simulink model "trajectoryReplay"  (R2018b)
settings: configuration reference "Physics" (kept outside this file)
StartFcn:
  | dictObj = Simulink.data.dictionary.open('ScenarioDefinition.sldd');
  | secObj = getSection(dictObj, 'Design Data');
  | enObj = getEntry(secObj, 'Raceline_Op1');
  | temp = getValue(enObj);
  | set_param('trajectoryReplay/max_v_Op1','Value',num2str(max(temp.vx_mps)));
  | 
  | close(dictObj);
  | clear dictObj secObj enObj temp;
model workspace (MAT data in the model file):
  F_N_Op = Simulink.Parameter
  F_N_Op.Value = [1 2 3 4 5 6 7 8 9 10 11 12 ... (5000 elements, 5000x1)]
  F_N_Op.DataType = 'auto'
  F_N_Op.Dimensions = [5000 1]
  ValidPointCnt_Op = 4844
  ax_mps2_Op = Simulink.Parameter
  ax_mps2_Op.Value = [1 2 3 4 5 6 7 8 9 10 11 12 ... (5000 elements, 5000x1)]
  ax_mps2_Op.DataType = 'auto'
  ax_mps2_Op.Dimensions = [5000 1]
  dPsi_radps = Simulink.Parameter
  dPsi_radps.Value = 0
  dPsi_radps.DataType = 'auto'
  dPsi_radps.Dimensions = [1 1]
  delta_rad_Op = Simulink.Parameter
  delta_rad_Op.Value = [1 2 3 4 5 6 7 8 9 10 11 12 ... (5000 elements, 5000x1)]
  delta_rad_Op.DataType = 'auto'
  delta_rad_Op.Dimensions = [5000 1]
  kappa_radpm_Op = Simulink.Parameter
  kappa_radpm_Op.Value = [1 2 3 4 5 6 7 8 9 10 11 12 ... (5000 elements, 5000x1)]
  kappa_radpm_Op.DataType = 'auto'
  kappa_radpm_Op.Dimensions = [5000 1]
  psi0_rad = Simulink.Parameter
  psi0_rad.Value = 0
  psi0_rad.DataType = 'auto'
  psi0_rad.Dimensions = [1 1]
  psi_rad = Simulink.Parameter
  psi_rad.Value = 0
  psi_rad.DataType = 'auto'
  psi_rad.Dimensions = [1 1]
  psi_rad_Op = Simulink.Parameter
  psi_rad_Op.Value = [1 2 3 4 5 6 7 8 9 10 11 12 ... (5000 elements, 5000x1)]
  psi_rad_Op.DataType = 'auto'
  psi_rad_Op.Dimensions = [5000 1]
  s0_m = Simulink.Parameter
  s0_m.Value = 0
  s0_m.DataType = 'auto'
  s0_m.Dimensions = [1 1]
  s_m_Op = Simulink.Parameter
  s_m_Op.Value = [1 2 3 4 5 6 7 8 9 10 11 12 ... (5000 elements, 5000x1)]
  s_m_Op.DataType = 'auto'
  s_m_Op.Dimensions = [5000 1]
  s_m_end_Op = Simulink.Parameter
  s_m_end_Op.Value = 0
  s_m_end_Op.DataType = 'double'
  s_m_end_Op.Dimensions = [1 1]
  velGain_Op = Simulink.Parameter
  velGain_Op.Value = 0
  velGain_Op.DataType = 'auto'
  velGain_Op.Dimensions = [1 1]
  vx_mps = Simulink.Parameter
  vx_mps.Value = 0
  vx_mps.DataType = 'auto'
  vx_mps.Dimensions = [1 1]
  vx_mps_Op = Simulink.Parameter
  vx_mps_Op.Value = [1 2 3 4 5 6 7 8 9 10 11 12 ... (5000 elements, 5000x1)]
  vx_mps_Op.DataType = 'auto'
  vx_mps_Op.Dimensions = [5000 1]
  vy_mps = Simulink.Parameter
  vy_mps.Value = 0
  vy_mps.DataType = 'auto'
  vy_mps.Dimensions = [1 1]
  x0_m = Simulink.Parameter
  x0_m.Value = 0
  x0_m.DataType = 'auto'
  x0_m.Dimensions = [1 1]
  x0_vehiclepose_Op = Simulink.Parameter
  x0_vehiclepose_Op.Value = [0 0 0]
  x0_vehiclepose_Op.DataType = 'double'
  x0_vehiclepose_Op.Dimensions = [1 3]
  x_m = Simulink.Parameter
  x_m.Value = 0
  x_m.DataType = 'double'
  x_m.Dimensions = [1 1]
  x_m_Op = Simulink.Parameter
  x_m_Op.Value = [1 2 3 4 5 6 7 8 9 10 11 12 ... (5000 elements, 5000x1)]
  x_m_Op.DataType = 'auto'
  x_m_Op.Dimensions = [5000 1]
  y0_m = Simulink.Parameter
  y0_m.Value = 0
  y0_m.DataType = 'auto'
  y0_m.Dimensions = [1 1]
  y_m = Simulink.Parameter
  y_m.Value = 0
  y_m.DataType = 'double'
  y_m.Dimensions = [1 1]
  y_m_Op = Simulink.Parameter
  y_m_Op.Value = [1 2 3 4 5 6 7 8 9 10 11 12 ... (5000 elements, 5000x1)]
  y_m_Op.DataType = 'auto'
  y_m_Op.Dimensions = [5000 1]
undefined symbols (not defined in the file): tSSlow
libraries: simulink x1
settings Model: DataDictionary=trajectoryReplay.sldd  ParameterArgumentNames=F_N_Op,ValidPointCnt_Op,ax_mps2_Op,delta_rad_Op,kappa_radpm_Op,psi_rad_Op,s0_m,s_m_Op,s_m_end_Op,velGain_Op,vx_mps_Op,x0_vehiclepose_Op,x_m_Op,y_m_Op  OrderedModelArguments=off  Creator=wischnewski  LastModifiedBy=ge34qer

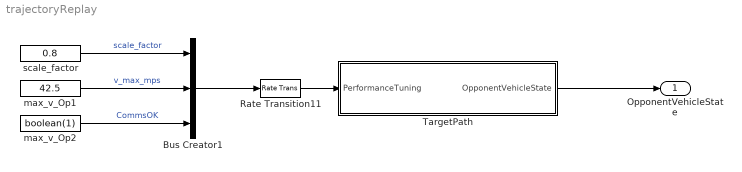
== system trajectoryReplay ==
  Bus Creator1 : BusCreator  Inputs=3  OutDataTypeStr=Bus: Planning_ControlPerformance_Feedback
  Rate Transition11 : RateTransition
  TargetPath : Subsystem  SystemSampleTime=tSSlow
  max_v_Op1 : Constant  Value=42.5
  max_v_Op2 : Constant  Value=boolean(1)
  scale_factor : Constant  Value=0.8
  OpponentVehicleState : Outport  OutDataTypeStr=Bus: V2X_Vehicle_Sim
  wires:
  Rate Transition11/1 -> TargetPath/1(PerformanceTuning)
  scale_factor/1 -> Bus Creator1/1  "scale_factor"
  max_v_Op1/1 -> Bus Creator1/2  "v_max_mps"
  Bus Creator1/1 -> Rate Transition11/1
  max_v_Op2/1 -> Bus Creator1/3  "CommsOK"
  TargetPath/1(OpponentVehicleState) -> OpponentVehicleState/1

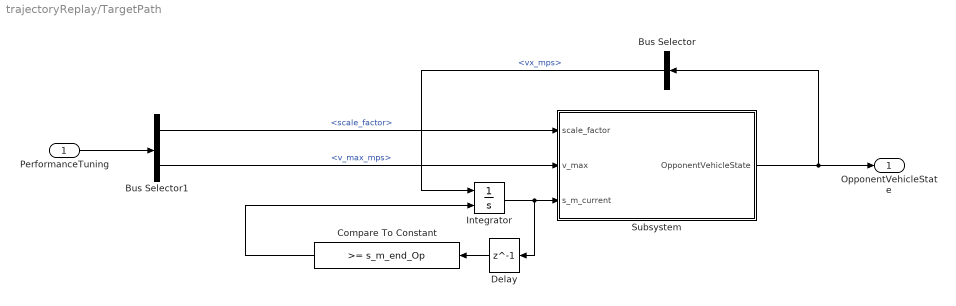
== system trajectoryReplay/TargetPath ==
  PerformanceTuning : Inport  OutDataTypeStr=Bus: Planning_ControlPerformance_Feedback
  Bus Selector : BusSelector  OutputSignals=vx_mps
  Bus Selector1 : BusSelector  OutputSignals=scale_factor,v_max_mps
  Compare To Constant : simulink/Logic and Bit Operations/Compare To Constant  relop=>=  const=s_m_end_Op  OutDataTypeStr=boolean
  Delay : Delay  DelayLength=1
  Integrator : Integrator  ExternalReset=rising  InitialCondition=s0_m
  Subsystem : Subsystem
  OpponentVehicleState : Outport
  wires:
  Integrator/1 -> Delay/1, Subsystem/3(s_m_current)
  Delay/1 -> Compare To Constant/1
  Subsystem/1(OpponentVehicleState) -> OpponentVehicleState/1, Bus Selector/1
  Compare To Constant/1 -> Integrator/2
  PerformanceTuning/1 -> Bus Selector1/1
  Bus Selector1/1 -> Subsystem/1(scale_factor)  "<scale_factor>"
  Bus Selector1/2 -> Subsystem/2(v_max)  "<v_max_mps>"
  Bus Selector/1 -> Integrator/1  "<vx_mps>"

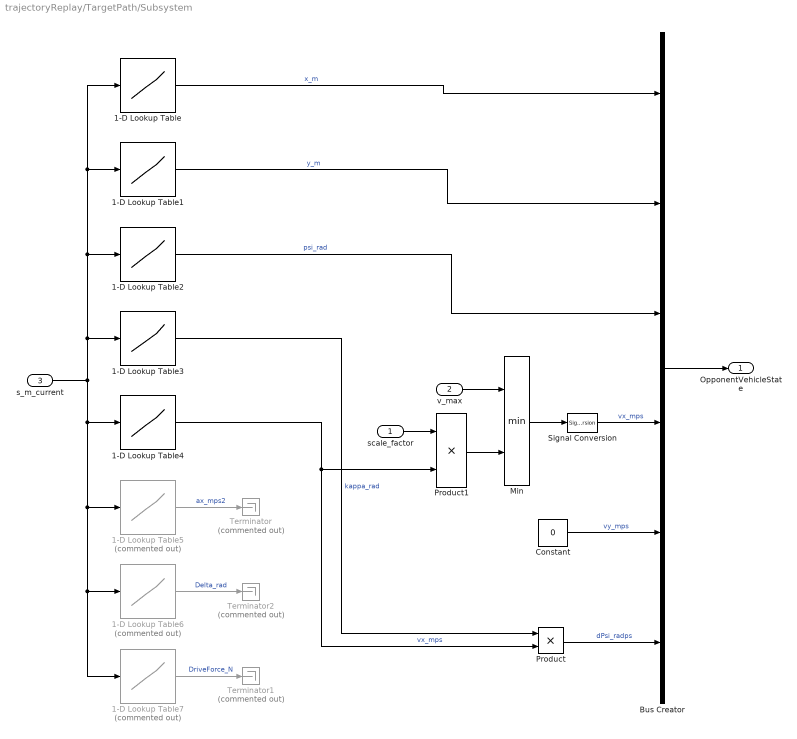
== system trajectoryReplay/TargetPath/Subsystem ==
  scale_factor : Inport
  v_max : Inport  Port=2
  s_m_current : Inport  Port=3
  1-D Lookup Table : Lookup_n-D  NumberOfTableDimensions=1  BreakpointsForDimension1=s_m_Op  Table=x_m_Op  InternalRulePriority=Speed  RndMeth=Simplest  InputSameDT=on
  1-D Lookup Table1 : Lookup_n-D  NumberOfTableDimensions=1  BreakpointsForDimension1=s_m_Op  Table=y_m_Op  InternalRulePriority=Speed  RndMeth=Simplest  InputSameDT=on
  1-D Lookup Table2 : Lookup_n-D  NumberOfTableDimensions=1  BreakpointsForDimension1=s_m_Op  Table=psi_rad_Op  InternalRulePriority=Speed  RndMeth=Simplest  InputSameDT=on
  1-D Lookup Table3 : Lookup_n-D  NumberOfTableDimensions=1  BreakpointsForDimension1=s_m_Op  Table=kappa_radpm_Op  InternalRulePriority=Speed  RndMeth=Simplest  InputSameDT=on
  1-D Lookup Table4 : Lookup_n-D  NumberOfTableDimensions=1  BreakpointsForDimension1=s_m_Op  Table=vx_mps_Op  InternalRulePriority=Speed  RndMeth=Simplest  InputSameDT=on
  1-D Lookup Table5 : Lookup_n-D  Commented=on  NumberOfTableDimensions=1  BreakpointsForDimension1=s_m_Op  Table=ax_mps2_Op  InternalRulePriority=Speed  RndMeth=Simplest  InputSameDT=on
  1-D Lookup Table6 : Lookup_n-D  Commented=on  NumberOfTableDimensions=1  BreakpointsForDimension1=s_m_Op  Table=delta_rad_Op  InternalRulePriority=Speed  RndMeth=Simplest  InputSameDT=on
  1-D Lookup Table7 : Lookup_n-D  Commented=on  NumberOfTableDimensions=1  BreakpointsForDimension1=s_m_Op  Table=F_N_Op  InternalRulePriority=Speed  RndMeth=Simplest  InputSameDT=on
  Bus Creator : BusCreator  Inputs=6  OutDataTypeStr=Bus: V2X_Vehicle_Sim
  Constant : Constant  Value=0
  Min : MinMax  Inputs=2
  Product : Product
  Product1 : Product
  Signal Conversion : SignalConversion  OverrideOpt=off
  Terminator : Terminator  Commented=on
  Terminator1 : Terminator  Commented=on
  Terminator2 : Terminator  Commented=on
  OpponentVehicleState : Outport
  wires:
  1-D Lookup Table6/1 -> Terminator2/1  "Delta_rad"
  1-D Lookup Table/1 -> Bus Creator/1  "x_m"
  s_m_current/1 -> 1-D Lookup Table/1, 1-D Lookup Table1/1, 1-D Lookup Table2/1, 1-D Lookup Table3/1, 1-D Lookup Table7/1, 1-D Lookup Table6/1, 1-D Lookup Table5/1, 1-D Lookup Table4/1
  1-D Lookup Table7/1 -> Terminator1/1  "DriveForce_N"
  1-D Lookup Table2/1 -> Bus Creator/3  "psi_rad"
  Bus Creator/1 -> OpponentVehicleState/1
  1-D Lookup Table1/1 -> Bus Creator/2  "y_m"
  1-D Lookup Table5/1 -> Terminator/1  "ax_mps2"
  1-D Lookup Table3/1 -> Product/1  "kappa_rad"
  1-D Lookup Table4/1 -> Product/2, Product1/2  "vx_mps"
  Constant/1 -> Bus Creator/5  "vy_mps"
  Product/1 -> Bus Creator/6  "dPsi_radps"
  Signal Conversion/1 -> Bus Creator/4  "vx_mps"
  Product1/1 -> Min/2
  Min/1 -> Signal Conversion/1
  scale_factor/1 -> Product1/1
  v_max/1 -> Min/1
